simulink model "clearing_faulted_segment_travelling_Wave"  (R2018a)
settings: Solver=ode23t  StartTime=0.0  StopTime=2  MaxStep=1e-3  RelTol=1e-3
values from neighbouring files (symbols this model uses):
  AC_lim = [1.5 -1.5]    [MT_HVDC_initialize.m]
  C_pm = 10.48e-3    (= 0.01048)    [MT_HVDC_initialize.m]
  ccsc_lim = [1.0 -1.0]    [MT_HVDC_initialize.m]
  DC_lim = [1.05 -1.05]    [MT_HVDC_initialize.m]
  f = 50    [MT_HVDC_initialize.m]
  Fc = 50    [MT_HVDC_initialize.m]
  Fn_filter = 1000    [MT_HVDC_initialize.m]
  Ireg_lim_i = [1.5, -1.5]    [MT_HVDC_initialize.m]
  Ireg_lim_r = [1.5, -1.5]    [MT_HVDC_initialize.m]
  Ki_ACreg_i = 260    [MT_HVDC_initialize.m]
  Ki_ccsc = 5    [MT_HVDC_initialize.m]
  Ki_DCreg_r = 150    [MT_HVDC_initialize.m]
  Ki_Ireg_i = 200    [MT_HVDC_initialize.m]
  Ki_Ireg_r = 100    [MT_HVDC_initialize.m]
  Ki_R_inv = 150000    [MT_HVDC_initialize.m]
  Ki_R_rec = 5000    [MT_HVDC_initialize.m]
  Kp_ACreg_i = 2    [MT_HVDC_initialize.m]
  Kp_ccsc = 1    [MT_HVDC_initialize.m]
  Kp_DCreg_r = 8    [MT_HVDC_initialize.m]
  Kp_Ireg_i = 2    [MT_HVDC_initialize.m]
  Kp_Ireg_r = 2    [MT_HVDC_initialize.m]
  Kp_R_inv = 0.001    [MT_HVDC_initialize.m]
  Kp_R_rec = 0.001    [MT_HVDC_initialize.m]
  L1_pu = 0.109    [MT_HVDC_initialize.m]
  L2_pu = 0.0824    [MT_HVDC_initialize.m]
  L_arm = L_arm_pu*Z_base66/w    [MT_HVDC_initialize.m]
  L_arm_pu = 0.15    [MT_HVDC_initialize.m]
  L_int = X_int/w    [MT_HVDC_initialize.m]
  n = 50    [MT_HVDC_initialize.m]
  n2 = 50    [MT_HVDC_initialize.m]
  P_nom = 220e6    (= 220000000)    [MT_HVDC_initialize.m]
  R1_pu = 0.00206    [MT_HVDC_initialize.m]
  R2_pu = 0.00206    [MT_HVDC_initialize.m]
  R_arm = 0.03    [MT_HVDC_initialize.m]
  R_arm_pu = R_arm/Z_base66    [MT_HVDC_initialize.m]
  R_int = sqrt((z_int_400^2)/(1+xr_ratio^2))    [MT_HVDC_initialize.m]
  Rg_T1 = 40    [MT_HVDC_initialize.m]
  S1_nom = P_nom    (= 220000000)    [MT_HVDC_initialize.m]
  S2_nom = P_nom    (= 220000000)    [MT_HVDC_initialize.m]
  T_fault = 1.4    [MT_HVDC_initialize.m]
  Ts_Control = 40e-6    (= 4e-05)    [MT_HVDC_initialize.m]
  Ts_Power = 20e-6    (= 2e-05)    [MT_HVDC_initialize.m]
  V1_prim = V_prim    (= 400000)    [MT_HVDC_initialize.m]
  V1_sec = V_grid    (= 66000)    [MT_HVDC_initialize.m]
  V2_prim = V_grid    (= 66000)    [MT_HVDC_initialize.m]
  V2_sec = 18e3    (= 18000)    [MT_HVDC_initialize.m]
  V_ac_ref = 1.035    [MT_HVDC_initialize.m]
  V_grid = 66e3    (= 66000)    [MT_HVDC_initialize.m]
  V_prim = 400e3    (= 400000)    [MT_HVDC_initialize.m]
  Vc_pm_r = 0*Vdc_nom/n    (= 0)    [MT_HVDC_initialize.m]
  Vdc_nom = 135e3    (= 135000)    [MT_HVDC_initialize.m]
  w = 2*pi*f    (= 314.159265359)    [MT_HVDC_initialize.m]
  z0z1 = 0.8    [MT_HVDC_initialize.m]
  Zeta_filter = 1    [MT_HVDC_initialize.m]
undefined symbols (not defined in the file or in its folder): D1, Delta, DiscIntNeverNeededParam
libraries: powerlib x417, powerlib_meascontrol x130, simulink x84, powerlib_extras x8, simulink_extras x5
(part 6 of 17)

== system clearing_faulted_segment_travelling_Wave/MMC Converter4 ==
  g : Inport
  Current Measurement{,1..5} (6 alike) : powerlib/Measurements/Current Measurement  PhasorSimulation=off  OutputType=Complex  PSBequivalent=0
      settings: SourceProductName=Simscape Electrical
  Demux : Demux  Outputs=6
  Half-Bridge MMC Ap : Subsystem  mask(Half-Bridge MMC - Aggregate Model){n=n, C=C_pm, Vc_Initial=Vc_pm_r, Ts=Ts_Power}
      mask prompts: n "Number of power modules"; C "Capacitor value (F):"; Vc_Initial "Capacitor initial voltage (V):"; Ts "Sample time (s):"
      mask help:
      | Implement a half-bridge Modular Multilevel Converter (MMC) using a switching-function model where only one equivalent module is used to represent all power modules.
      |
      | The control signal is a two-element vector [ Nin, Nbl ], where Nin represents the number of inserted modules and Nbl represents the number of modules in the blocked-state. The output Vc (capacitor voltage) has only one element and gives the average value of the capacitors modules.
      |
      | With this aggregate model, it is assumed that capacitor voltage of all power modules are well-balanced. However, control system dynamics, converter harmonics content and circulating currents phenomena are all-well represented. The model runs a lot faster than the detailed model which uses two switching devices and one capacitor for each individual power module. This aggregate model is also well-suited for real-time simulation.
      settings: AttributesFormatString=(Aggregate model of %<n> PM)
      mask Display:
      | x1=0.0;
      | plot([0.17 0.5]+x1,[0.93 0.93])
      | plot([0.5 0.5]+x1,[0.93,0.80])
      | plot([0.5 0.38]+x1,[0.80 0.74])
      | plot([0.38 0.38]+x1,[0.80 0.62])
      | plot([0.38 0.5]+x1,[0.68 0.62])
      | plot([0.5 0.5]+x1,[0.62 0.52])
      | plot([0.45 0.5 0.43]+x1,[0.68 0.62 0.60])
      | %
      | y1=0.40-0.03;
      | plot([0.5 0.5]+x1,[0.93,0.80]-y1)
      | plot([0.5 0.38]+x1,[0.80 0.74]-y1)
      | plot([0.38 0.38]+x1,[0.80 0.62]-y1)
      | plot([0.38 0.5]+x1,[0.68 0.62]-y1)
      | plot([0.5 0.5]+x1,[0.62 0.52]-y1)
      | plot([0.45 0.5 0.43]+x1,[0.68 0.62 0.60]-y1)
      | plot([0.5 0.5]+x1,[0.2,0.10])
      | plot([0.17 0.5]+x1,[0.1 0.1])
      | %
      | plot([0.5 0.6]+x1,[0.84 0.84]+0.03)
      | plot([0.6 0.6]+x1,[0.84 0.74]+0.03)
      | plot([0.6 0.56]+x1,[0.74 0.69]+0.03)
      | plot([0.6 0.64]+x1,[0.74 0.69]+0.03)
      | plot([0.56 0.64]+x1,[0.69 0.69]+0.03)
      | plot([0.6 0.6]+x1,[0.69 0.57]+0.03)
      | plot([0.5 0.6]+x1,[0.57 0.57]+0.03)
      | plot([0.55 0.65]+x1,[0.74 0.74]+0.03)
      | %
      | y2=0.4-0.03;
      | plot([0.5 0.6]+x1,[0.84 0.84]-y2)
      | plot([0.6 0.6]+x1,[0.84 0.74]-y2)
      | plot([0.6 0.56]+x1,[0.74 0.69]-y2)
      | plot([0.6 0.64]+x1,[0.74 0.69]-y2)
      | plot([0.56 0.64]+x1,[0.69 0.69]-y2)
      | plot([0.6 0.6]+x1,[0.69 0.57]-y2)
      | plot([0.5 0.6]+x1,[0.57 0.57]-y2)
      | plot([0.55 0.65]+x1,[0.74 0.74]-y2)
      | %
      | plot([0.5 0.75]+x1,[0.53 0.53])
      | plot([0.75 0.75]+x1,[0.53 0.57])
      | plot([0.75 0.75]+x1,[0.61 0.65])
      | plot([0.75 0.75]+x1,[0.69 0.73])
      | plot([0.75 0.75]+x1,[0.77 0.81])
      | plot([0.75 0.75]+x1,[0.09 0.07])
      | plot([0.75 0.75]+x1,[0.04 0.01])
      | %
      | plot([0.34 0.34]+x1,[0.65 0.75])
      | plot([0.28 0.34]+x1,[0.7 0.7])
      | %
      | plot([0.34 0.34]+x1,[0.65 0.75]-y2)
      | plot([0.28 0.34]+x1,[0.7 0.7]-y2)
      | %
      | %Capacitor
      | plot([0.16 0.16],[0.93 0.54])
      | plot([0.16 0.16],[0.47 0.10])
      | plot([0.04 0.27],[0.54 0.54])
      | plot([0.04 0.27],[0.47 0.47])
      | %
      | plot([0.5 0.75],[0.1 0.1])
      | % text(0.78,0.5,'1')
      | % text(0.78,0.12,'2')
      | %
      | color('blue')
      | port_label('input',1,'N')
  Half-Bridge MMC Ap1 : Subsystem  mask(Half-Bridge MMC - Aggregate Model){n=n, C=C_pm, Vc_Initial=Vc_pm_r, Ts=Ts_Power}
      mask prompts: n "Number of power modules"; C "Capacitor value (F):"; Vc_Initial "Capacitor initial voltage (V):"; Ts "Sample time (s):"
      mask help:
      | Implement a half-bridge Modular Multilevel Converter (MMC) using a switching-function model where only one equivalent module is used to represent all power modules.
      |
      | The control signal is a two-element vector [ Nin, Nbl ], where Nin represents the number of inserted modules and Nbl represents the number of modules in the blocked-state. The output Vc (capacitor voltage) has only one element and gives the average value of the capacitors modules.
      |
      | With this aggregate model, it is assumed that capacitor voltage of all power modules are well-balanced. However, control system dynamics, converter harmonics content and circulating currents phenomena are all-well represented. The model runs a lot faster than the detailed model which uses two switching devices and one capacitor for each individual power module. This aggregate model is also well-suited for real-time simulation.
      settings: AttributesFormatString=(Aggregate model of %<n> PM)
      mask Display:
      | x1=0.0;
      | plot([0.17 0.5]+x1,[0.93 0.93])
      | plot([0.5 0.5]+x1,[0.93,0.80])
      | plot([0.5 0.38]+x1,[0.80 0.74])
      | plot([0.38 0.38]+x1,[0.80 0.62])
      | plot([0.38 0.5]+x1,[0.68 0.62])
      | plot([0.5 0.5]+x1,[0.62 0.52])
      | plot([0.45 0.5 0.43]+x1,[0.68 0.62 0.60])
      | %
      | y1=0.40-0.03;
      | plot([0.5 0.5]+x1,[0.93,0.80]-y1)
      | plot([0.5 0.38]+x1,[0.80 0.74]-y1)
      | plot([0.38 0.38]+x1,[0.80 0.62]-y1)
      | plot([0.38 0.5]+x1,[0.68 0.62]-y1)
      | plot([0.5 0.5]+x1,[0.62 0.52]-y1)
      | plot([0.45 0.5 0.43]+x1,[0.68 0.62 0.60]-y1)
      | plot([0.5 0.5]+x1,[0.2,0.10])
      | plot([0.17 0.5]+x1,[0.1 0.1])
      | %
      | plot([0.5 0.6]+x1,[0.84 0.84]+0.03)
      | plot([0.6 0.6]+x1,[0.84 0.74]+0.03)
      | plot([0.6 0.56]+x1,[0.74 0.69]+0.03)
      | plot([0.6 0.64]+x1,[0.74 0.69]+0.03)
      | plot([0.56 0.64]+x1,[0.69 0.69]+0.03)
      | plot([0.6 0.6]+x1,[0.69 0.57]+0.03)
      | plot([0.5 0.6]+x1,[0.57 0.57]+0.03)
      | plot([0.55 0.65]+x1,[0.74 0.74]+0.03)
      | %
      | y2=0.4-0.03;
      | plot([0.5 0.6]+x1,[0.84 0.84]-y2)
      | plot([0.6 0.6]+x1,[0.84 0.74]-y2)
      | plot([0.6 0.56]+x1,[0.74 0.69]-y2)
      | plot([0.6 0.64]+x1,[0.74 0.69]-y2)
      | plot([0.56 0.64]+x1,[0.69 0.69]-y2)
      | plot([0.6 0.6]+x1,[0.69 0.57]-y2)
      | plot([0.5 0.6]+x1,[0.57 0.57]-y2)
      | plot([0.55 0.65]+x1,[0.74 0.74]-y2)
      | %
      | plot([0.5 0.75]+x1,[0.53 0.53])
      | plot([0.75 0.75]+x1,[0.53 0.57])
      | plot([0.75 0.75]+x1,[0.61 0.65])
      | plot([0.75 0.75]+x1,[0.69 0.73])
      | plot([0.75 0.75]+x1,[0.77 0.81])
      | plot([0.75 0.75]+x1,[0.09 0.07])
      | plot([0.75 0.75]+x1,[0.04 0.01])
      | %
      | plot([0.34 0.34]+x1,[0.65 0.75])
      | plot([0.28 0.34]+x1,[0.7 0.7])
      | %
      | plot([0.34 0.34]+x1,[0.65 0.75]-y2)
      | plot([0.28 0.34]+x1,[0.7 0.7]-y2)
      | %
      | %Capacitor
      | plot([0.16 0.16],[0.93 0.54])
      | plot([0.16 0.16],[0.47 0.10])
      | plot([0.04 0.27],[0.54 0.54])
      | plot([0.04 0.27],[0.47 0.47])
      | %
      | plot([0.5 0.75],[0.1 0.1])
      | % text(0.78,0.5,'1')
      | % text(0.78,0.12,'2')
      | %
      | color('blue')
      | port_label('input',1,'N')
  Half-Bridge MMC Ap2 : Subsystem  mask(Half-Bridge MMC - Aggregate Model){n=n, C=C_pm, Vc_Initial=Vc_pm_r, Ts=Ts_Power}
      mask prompts: n "Number of power modules"; C "Capacitor value (F):"; Vc_Initial "Capacitor initial voltage (V):"; Ts "Sample time (s):"
      mask help:
      | Implement a half-bridge Modular Multilevel Converter (MMC) using a switching-function model where only one equivalent module is used to represent all power modules.
      |
      | The control signal is a two-element vector [ Nin, Nbl ], where Nin represents the number of inserted modules and Nbl represents the number of modules in the blocked-state. The output Vc (capacitor voltage) has only one element and gives the average value of the capacitors modules.
      |
      | With this aggregate model, it is assumed that capacitor voltage of all power modules are well-balanced. However, control system dynamics, converter harmonics content and circulating currents phenomena are all-well represented. The model runs a lot faster than the detailed model which uses two switching devices and one capacitor for each individual power module. This aggregate model is also well-suited for real-time simulation.
      settings: AttributesFormatString=(Aggregate model of %<n> PM)
      mask Display:
      | x1=0.0;
      | plot([0.17 0.5]+x1,[0.93 0.93])
      | plot([0.5 0.5]+x1,[0.93,0.80])
      | plot([0.5 0.38]+x1,[0.80 0.74])
      | plot([0.38 0.38]+x1,[0.80 0.62])
      | plot([0.38 0.5]+x1,[0.68 0.62])
      | plot([0.5 0.5]+x1,[0.62 0.52])
      | plot([0.45 0.5 0.43]+x1,[0.68 0.62 0.60])
      | %
      | y1=0.40-0.03;
      | plot([0.5 0.5]+x1,[0.93,0.80]-y1)
      | plot([0.5 0.38]+x1,[0.80 0.74]-y1)
      | plot([0.38 0.38]+x1,[0.80 0.62]-y1)
      | plot([0.38 0.5]+x1,[0.68 0.62]-y1)
      | plot([0.5 0.5]+x1,[0.62 0.52]-y1)
      | plot([0.45 0.5 0.43]+x1,[0.68 0.62 0.60]-y1)
      | plot([0.5 0.5]+x1,[0.2,0.10])
      | plot([0.17 0.5]+x1,[0.1 0.1])
      | %
      | plot([0.5 0.6]+x1,[0.84 0.84]+0.03)
      | plot([0.6 0.6]+x1,[0.84 0.74]+0.03)
      | plot([0.6 0.56]+x1,[0.74 0.69]+0.03)
      | plot([0.6 0.64]+x1,[0.74 0.69]+0.03)
      | plot([0.56 0.64]+x1,[0.69 0.69]+0.03)
      | plot([0.6 0.6]+x1,[0.69 0.57]+0.03)
      | plot([0.5 0.6]+x1,[0.57 0.57]+0.03)
      | plot([0.55 0.65]+x1,[0.74 0.74]+0.03)
      | %
      | y2=0.4-0.03;
      | plot([0.5 0.6]+x1,[0.84 0.84]-y2)
      | plot([0.6 0.6]+x1,[0.84 0.74]-y2)
      | plot([0.6 0.56]+x1,[0.74 0.69]-y2)
      | plot([0.6 0.64]+x1,[0.74 0.69]-y2)
      | plot([0.56 0.64]+x1,[0.69 0.69]-y2)
      | plot([0.6 0.6]+x1,[0.69 0.57]-y2)
      | plot([0.5 0.6]+x1,[0.57 0.57]-y2)
      | plot([0.55 0.65]+x1,[0.74 0.74]-y2)
      | %
      | plot([0.5 0.75]+x1,[0.53 0.53])
      | plot([0.75 0.75]+x1,[0.53 0.57])
      | plot([0.75 0.75]+x1,[0.61 0.65])
      | plot([0.75 0.75]+x1,[0.69 0.73])
      | plot([0.75 0.75]+x1,[0.77 0.81])
      | plot([0.75 0.75]+x1,[0.09 0.07])
      | plot([0.75 0.75]+x1,[0.04 0.01])
      | %
      | plot([0.34 0.34]+x1,[0.65 0.75])
      | plot([0.28 0.34]+x1,[0.7 0.7])
      | %
      | plot([0.34 0.34]+x1,[0.65 0.75]-y2)
      | plot([0.28 0.34]+x1,[0.7 0.7]-y2)
      | %
      | %Capacitor
      | plot([0.16 0.16],[0.93 0.54])
      | plot([0.16 0.16],[0.47 0.10])
      | plot([0.04 0.27],[0.54 0.54])
      | plot([0.04 0.27],[0.47 0.47])
      | %
      | plot([0.5 0.75],[0.1 0.1])
      | % text(0.78,0.5,'1')
      | % text(0.78,0.12,'2')
      | %
      | color('blue')
      | port_label('input',1,'N')
  Half-Bridge MMC Ap3 : Subsystem  mask(Half-Bridge MMC - Aggregate Model){n=n, C=C_pm, Vc_Initial=Vc_pm_r, Ts=Ts_Power}
      mask prompts: n "Number of power modules"; C "Capacitor value (F):"; Vc_Initial "Capacitor initial voltage (V):"; Ts "Sample time (s):"
      mask help:
      | Implement a half-bridge Modular Multilevel Converter (MMC) using a switching-function model where only one equivalent module is used to represent all power modules.
      |
      | The control signal is a two-element vector [ Nin, Nbl ], where Nin represents the number of inserted modules and Nbl represents the number of modules in the blocked-state. The output Vc (capacitor voltage) has only one element and gives the average value of the capacitors modules.
      |
      | With this aggregate model, it is assumed that capacitor voltage of all power modules are well-balanced. However, control system dynamics, converter harmonics content and circulating currents phenomena are all-well represented. The model runs a lot faster than the detailed model which uses two switching devices and one capacitor for each individual power module. This aggregate model is also well-suited for real-time simulation.
      settings: AttributesFormatString=(Aggregate model of %<n> PM)
      mask Display:
      | x1=0.0;
      | plot([0.17 0.5]+x1,[0.93 0.93])
      | plot([0.5 0.5]+x1,[0.93,0.80])
      | plot([0.5 0.38]+x1,[0.80 0.74])
      | plot([0.38 0.38]+x1,[0.80 0.62])
      | plot([0.38 0.5]+x1,[0.68 0.62])
      | plot([0.5 0.5]+x1,[0.62 0.52])
      | plot([0.45 0.5 0.43]+x1,[0.68 0.62 0.60])
      | %
      | y1=0.40-0.03;
      | plot([0.5 0.5]+x1,[0.93,0.80]-y1)
      | plot([0.5 0.38]+x1,[0.80 0.74]-y1)
      | plot([0.38 0.38]+x1,[0.80 0.62]-y1)
      | plot([0.38 0.5]+x1,[0.68 0.62]-y1)
      | plot([0.5 0.5]+x1,[0.62 0.52]-y1)
      | plot([0.45 0.5 0.43]+x1,[0.68 0.62 0.60]-y1)
      | plot([0.5 0.5]+x1,[0.2,0.10])
      | plot([0.17 0.5]+x1,[0.1 0.1])
      | %
      | plot([0.5 0.6]+x1,[0.84 0.84]+0.03)
      | plot([0.6 0.6]+x1,[0.84 0.74]+0.03)
      | plot([0.6 0.56]+x1,[0.74 0.69]+0.03)
      | plot([0.6 0.64]+x1,[0.74 0.69]+0.03)
      | plot([0.56 0.64]+x1,[0.69 0.69]+0.03)
      | plot([0.6 0.6]+x1,[0.69 0.57]+0.03)
      | plot([0.5 0.6]+x1,[0.57 0.57]+0.03)
      | plot([0.55 0.65]+x1,[0.74 0.74]+0.03)
      | %
      | y2=0.4-0.03;
      | plot([0.5 0.6]+x1,[0.84 0.84]-y2)
      | plot([0.6 0.6]+x1,[0.84 0.74]-y2)
      | plot([0.6 0.56]+x1,[0.74 0.69]-y2)
      | plot([0.6 0.64]+x1,[0.74 0.69]-y2)
      | plot([0.56 0.64]+x1,[0.69 0.69]-y2)
      | plot([0.6 0.6]+x1,[0.69 0.57]-y2)
      | plot([0.5 0.6]+x1,[0.57 0.57]-y2)
      | plot([0.55 0.65]+x1,[0.74 0.74]-y2)
      | %
      | plot([0.5 0.75]+x1,[0.53 0.53])
      | plot([0.75 0.75]+x1,[0.53 0.57])
      | plot([0.75 0.75]+x1,[0.61 0.65])
      | plot([0.75 0.75]+x1,[0.69 0.73])
      | plot([0.75 0.75]+x1,[0.77 0.81])
      | plot([0.75 0.75]+x1,[0.09 0.07])
      | plot([0.75 0.75]+x1,[0.04 0.01])
      | %
      | plot([0.34 0.34]+x1,[0.65 0.75])
      | plot([0.28 0.34]+x1,[0.7 0.7])
      | %
      | plot([0.34 0.34]+x1,[0.65 0.75]-y2)
      | plot([0.28 0.34]+x1,[0.7 0.7]-y2)
      | %
      | %Capacitor
      | plot([0.16 0.16],[0.93 0.54])
      | plot([0.16 0.16],[0.47 0.10])
      | plot([0.04 0.27],[0.54 0.54])
      | plot([0.04 0.27],[0.47 0.47])
      | %
      | plot([0.5 0.75],[0.1 0.1])
      | % text(0.78,0.5,'1')
      | % text(0.78,0.12,'2')
      | %
      | color('blue')
      | port_label('input',1,'N')
  Half-Bridge MMC Ap4 : Subsystem  mask(Half-Bridge MMC - Aggregate Model){n=n, C=C_pm, Vc_Initial=Vc_pm_r, Ts=Ts_Power}
      mask prompts: n "Number of power modules"; C "Capacitor value (F):"; Vc_Initial "Capacitor initial voltage (V):"; Ts "Sample time (s):"
      mask help:
      | Implement a half-bridge Modular Multilevel Converter (MMC) using a switching-function model where only one equivalent module is used to represent all power modules.
      |
      | The control signal is a two-element vector [ Nin, Nbl ], where Nin represents the number of inserted modules and Nbl represents the number of modules in the blocked-state. The output Vc (capacitor voltage) has only one element and gives the average value of the capacitors modules.
      |
      | With this aggregate model, it is assumed that capacitor voltage of all power modules are well-balanced. However, control system dynamics, converter harmonics content and circulating currents phenomena are all-well represented. The model runs a lot faster than the detailed model which uses two switching devices and one capacitor for each individual power module. This aggregate model is also well-suited for real-time simulation.
      settings: AttributesFormatString=(Aggregate model of %<n> PM)
      mask Display:
      | x1=0.0;
      | plot([0.17 0.5]+x1,[0.93 0.93])
      | plot([0.5 0.5]+x1,[0.93,0.80])
      | plot([0.5 0.38]+x1,[0.80 0.74])
      | plot([0.38 0.38]+x1,[0.80 0.62])
      | plot([0.38 0.5]+x1,[0.68 0.62])
      | plot([0.5 0.5]+x1,[0.62 0.52])
      | plot([0.45 0.5 0.43]+x1,[0.68 0.62 0.60])
      | %
      | y1=0.40-0.03;
      | plot([0.5 0.5]+x1,[0.93,0.80]-y1)
      | plot([0.5 0.38]+x1,[0.80 0.74]-y1)
      | plot([0.38 0.38]+x1,[0.80 0.62]-y1)
      | plot([0.38 0.5]+x1,[0.68 0.62]-y1)
      | plot([0.5 0.5]+x1,[0.62 0.52]-y1)
      | plot([0.45 0.5 0.43]+x1,[0.68 0.62 0.60]-y1)
      | plot([0.5 0.5]+x1,[0.2,0.10])
      | plot([0.17 0.5]+x1,[0.1 0.1])
      | %
      | plot([0.5 0.6]+x1,[0.84 0.84]+0.03)
      | plot([0.6 0.6]+x1,[0.84 0.74]+0.03)
      | plot([0.6 0.56]+x1,[0.74 0.69]+0.03)
      | plot([0.6 0.64]+x1,[0.74 0.69]+0.03)
      | plot([0.56 0.64]+x1,[0.69 0.69]+0.03)
      | plot([0.6 0.6]+x1,[0.69 0.57]+0.03)
      | plot([0.5 0.6]+x1,[0.57 0.57]+0.03)
      | plot([0.55 0.65]+x1,[0.74 0.74]+0.03)
      | %
      | y2=0.4-0.03;
      | plot([0.5 0.6]+x1,[0.84 0.84]-y2)
      | plot([0.6 0.6]+x1,[0.84 0.74]-y2)
      | plot([0.6 0.56]+x1,[0.74 0.69]-y2)
      | plot([0.6 0.64]+x1,[0.74 0.69]-y2)
      | plot([0.56 0.64]+x1,[0.69 0.69]-y2)
      | plot([0.6 0.6]+x1,[0.69 0.57]-y2)
      | plot([0.5 0.6]+x1,[0.57 0.57]-y2)
      | plot([0.55 0.65]+x1,[0.74 0.74]-y2)
      | %
      | plot([0.5 0.75]+x1,[0.53 0.53])
      | plot([0.75 0.75]+x1,[0.53 0.57])
      | plot([0.75 0.75]+x1,[0.61 0.65])
      | plot([0.75 0.75]+x1,[0.69 0.73])
      | plot([0.75 0.75]+x1,[0.77 0.81])
      | plot([0.75 0.75]+x1,[0.09 0.07])
      | plot([0.75 0.75]+x1,[0.04 0.01])
      | %
      | plot([0.34 0.34]+x1,[0.65 0.75])
      | plot([0.28 0.34]+x1,[0.7 0.7])
      | %
      | plot([0.34 0.34]+x1,[0.65 0.75]-y2)
      | plot([0.28 0.34]+x1,[0.7 0.7]-y2)
      | %
      | %Capacitor
      | plot([0.16 0.16],[0.93 0.54])
      | plot([0.16 0.16],[0.47 0.10])
      | plot([0.04 0.27],[0.54 0.54])
      | plot([0.04 0.27],[0.47 0.47])
      | %
      | plot([0.5 0.75],[0.1 0.1])
      | % text(0.78,0.5,'1')
      | % text(0.78,0.12,'2')
      | %
      | color('blue')
      | port_label('input',1,'N')
  Half-Bridge MMC Ap5 : Subsystem  mask(Half-Bridge MMC - Aggregate Model){n=n, C=C_pm, Vc_Initial=Vc_pm_r, Ts=Ts_Power}
      mask prompts: n "Number of power modules"; C "Capacitor value (F):"; Vc_Initial "Capacitor initial voltage (V):"; Ts "Sample time (s):"
      mask help:
      | Implement a half-bridge Modular Multilevel Converter (MMC) using a switching-function model where only one equivalent module is used to represent all power modules.
      |
      | The control signal is a two-element vector [ Nin, Nbl ], where Nin represents the number of inserted modules and Nbl represents the number of modules in the blocked-state. The output Vc (capacitor voltage) has only one element and gives the average value of the capacitors modules.
      |
      | With this aggregate model, it is assumed that capacitor voltage of all power modules are well-balanced. However, control system dynamics, converter harmonics content and circulating currents phenomena are all-well represented. The model runs a lot faster than the detailed model which uses two switching devices and one capacitor for each individual power module. This aggregate model is also well-suited for real-time simulation.
      settings: AttributesFormatString=(Aggregate model of %<n> PM)
      mask Display:
      | x1=0.0;
      | plot([0.17 0.5]+x1,[0.93 0.93])
      | plot([0.5 0.5]+x1,[0.93,0.80])
      | plot([0.5 0.38]+x1,[0.80 0.74])
      | plot([0.38 0.38]+x1,[0.80 0.62])
      | plot([0.38 0.5]+x1,[0.68 0.62])
      | plot([0.5 0.5]+x1,[0.62 0.52])
      | plot([0.45 0.5 0.43]+x1,[0.68 0.62 0.60])
      | %
      | y1=0.40-0.03;
      | plot([0.5 0.5]+x1,[0.93,0.80]-y1)
      | plot([0.5 0.38]+x1,[0.80 0.74]-y1)
      | plot([0.38 0.38]+x1,[0.80 0.62]-y1)
      | plot([0.38 0.5]+x1,[0.68 0.62]-y1)
      | plot([0.5 0.5]+x1,[0.62 0.52]-y1)
      | plot([0.45 0.5 0.43]+x1,[0.68 0.62 0.60]-y1)
      | plot([0.5 0.5]+x1,[0.2,0.10])
      | plot([0.17 0.5]+x1,[0.1 0.1])
      | %
      | plot([0.5 0.6]+x1,[0.84 0.84]+0.03)
      | plot([0.6 0.6]+x1,[0.84 0.74]+0.03)
      | plot([0.6 0.56]+x1,[0.74 0.69]+0.03)
      | plot([0.6 0.64]+x1,[0.74 0.69]+0.03)
      | plot([0.56 0.64]+x1,[0.69 0.69]+0.03)
      | plot([0.6 0.6]+x1,[0.69 0.57]+0.03)
      | plot([0.5 0.6]+x1,[0.57 0.57]+0.03)
      | plot([0.55 0.65]+x1,[0.74 0.74]+0.03)
      | %
      | y2=0.4-0.03;
      | plot([0.5 0.6]+x1,[0.84 0.84]-y2)
      | plot([0.6 0.6]+x1,[0.84 0.74]-y2)
      | plot([0.6 0.56]+x1,[0.74 0.69]-y2)
      | plot([0.6 0.64]+x1,[0.74 0.69]-y2)
      | plot([0.56 0.64]+x1,[0.69 0.69]-y2)
      | plot([0.6 0.6]+x1,[0.69 0.57]-y2)
      | plot([0.5 0.6]+x1,[0.57 0.57]-y2)
      | plot([0.55 0.65]+x1,[0.74 0.74]-y2)
      | %
      | plot([0.5 0.75]+x1,[0.53 0.53])
      | plot([0.75 0.75]+x1,[0.53 0.57])
      | plot([0.75 0.75]+x1,[0.61 0.65])
      | plot([0.75 0.75]+x1,[0.69 0.73])
      | plot([0.75 0.75]+x1,[0.77 0.81])
      | plot([0.75 0.75]+x1,[0.09 0.07])
      | plot([0.75 0.75]+x1,[0.04 0.01])
      | %
      | plot([0.34 0.34]+x1,[0.65 0.75])
      | plot([0.28 0.34]+x1,[0.7 0.7])
      | %
      | plot([0.34 0.34]+x1,[0.65 0.75]-y2)
      | plot([0.28 0.34]+x1,[0.7 0.7]-y2)
      | %
      | %Capacitor
      | plot([0.16 0.16],[0.93 0.54])
      | plot([0.16 0.16],[0.47 0.10])
      | plot([0.04 0.27],[0.54 0.54])
      | plot([0.04 0.27],[0.47 0.47])
      | %
      | plot([0.5 0.75],[0.1 0.1])
      | % text(0.78,0.5,'1')
      | % text(0.78,0.12,'2')
      | %
      | color('blue')
      | port_label('input',1,'N')
  Mux : Mux  Inputs=6
  Mux1 : Mux  Inputs=6
  Series RLC Branch1 : powerlib/Elements/Series RLC Branch  LConnTagsString=__new0  RConnTagsString=__new0  BranchType=L  Resistance=R_arm  Inductance=L_arm  SetiL0=off  InitialCurrent=0  Capacitance=1e-6  Setx0=off  InitialVoltage=0  Measurements=None
      settings: SourceProductName=Simscape Electrical
  Series RLC Branch{2..6} (5 alike) : powerlib/Elements/Series RLC Branch  LConnTagsString=__new0  RConnTagsString=__new0  BranchType=RL  Resistance=R_arm  Inductance=L_arm  SetiL0=off  InitialCurrent=0  Capacitance=1e-6  Setx0=off  InitialVoltage=0  Measurements=None
      settings: SourceProductName=Simscape Electrical
  Series RLC Branch7 : powerlib/Elements/Series RLC Branch  LConnTagsString=__new0  RConnTagsString=__new0  BranchType=R  Resistance=R_arm  Inductance=L_arm  SetiL0=off  InitialCurrent=0  Capacitance=1e-6  Setx0=off  InitialVoltage=0  Measurements=None
      settings: SourceProductName=Simscape Electrical
  V_a : PMIOPort  Tag=PMCPort  Side=Left
  V_b : PMIOPort  Tag=PMCPort  Port=2  Side=Left
  V_c : PMIOPort  Tag=PMCPort  Port=3  Side=Left
  Vdc + : PMIOPort  Tag=PMCPort  Port=4  Side=Right
  Vdc - : PMIOPort  Tag=PMCPort  Port=5  Side=Right
  Vc : Outport
  I_arm : Outport  Port=2
  wires:
  Demux/6 -> [g6]
  Demux/5 -> [g5]
  Demux/4 -> [g4]
  Demux/3 -> [g3]
  Demux/2 -> [g2]
  Demux/1 -> [g1]
  Half-Bridge MMC Ap/1(Vc) -> [Vc1]
  Half-Bridge MMC Ap5/1(Vc) -> [Vc6]
  Half-Bridge MMC Ap3/1(Vc) -> [Vc2]
  Half-Bridge MMC Ap4/1(Vc) -> [Vc5]
  [Icu] -> Mux1/5
  [Ibl] -> Mux1/4
  [Icl] -> Mux1/6
  [Ial] -> Mux1/2
  [Iau] -> Mux1/1
  Mux1/1 -> I_arm/1
  [Ibu] -> Mux1/3
  Current Measurement2/1 -> [Ibu]
  Current Measurement5/1 -> [Icl]
  Current Measurement3/1 -> [Icu]
  Current Measurement4/1 -> [Ibl]
  Current Measurement/1 -> [Iau]
  Current Measurement1/1 -> [Ial]
  [Vc5] -> Mux/5
  Mux/1 -> Vc/1
  [Vc4] -> Mux/4
  [Vc1] -> Mux/1
  [Vc6] -> Mux/6
  [Vc3] -> Mux/3
  [g5] -> Half-Bridge MMC Ap1/1(g)
  [g1] -> Half-Bridge MMC Ap/1(g)
  [g4] -> Half-Bridge MMC Ap3/1(g)
  [g3] -> Half-Bridge MMC Ap4/1(g)
  [g2] -> Half-Bridge MMC Ap2/1(g)
  [g6] -> Half-Bridge MMC Ap5/1(g)
  g/1 -> Demux/1
  [Vc2] -> Mux/2
  Half-Bridge MMC Ap1/1(Vc) -> [Vc4]
  Half-Bridge MMC Ap2/1(Vc) -> [Vc3]
  connections:
  Half-Bridge MMC Ap1/LConn1 -- Current Measurement4/RConn1
  Half-Bridge MMC Ap5/LConn1 -- Current Measurement5/RConn1
  Half-Bridge MMC Ap2/LConn2 -- Current Measurement2/LConn1
  Half-Bridge MMC Ap4/LConn2 -- Current Measurement3/LConn1
  Vdc -/RConn1 -- Half-Bridge MMC Ap3/LConn2 -- Half-Bridge MMC Ap5/LConn2 -- Half-Bridge MMC Ap1/LConn2
  Half-Bridge MMC Ap3/LConn1 -- Current Measurement1/RConn1
  V_b/RConn1 -- Series RLC Branch2/RConn1 -- Series RLC Branch4/LConn1
  Series RLC Branch1/LConn1 -- Series RLC Branch7/RConn1
  Series RLC Branch3/RConn1 -- Current Measurement1/LConn1
  V_c/RConn1 -- Series RLC Branch5/LConn1 -- Series RLC Branch6/RConn1
  V_a/RConn1 -- Series RLC Branch1/RConn1 -- Series RLC Branch3/LConn1
  Series RLC Branch2/LConn1 -- Current Measurement2/RConn1
  Series RLC Branch4/RConn1 -- Current Measurement4/LConn1
  Current Measurement5/LConn1 -- Series RLC Branch5/RConn1
  Series RLC Branch6/LConn1 -- Current Measurement3/RConn1
  Vdc +/RConn1 -- Half-Bridge MMC Ap/LConn1 -- Half-Bridge MMC Ap4/LConn1 -- Half-Bridge MMC Ap2/LConn1
  Current Measurement/LConn1 -- Half-Bridge MMC Ap/LConn2
  Series RLC Branch7/LConn1 -- Current Measurement/RConn1

== system clearing_faulted_segment_travelling_Wave/Model Information ==
  note: References
      | [1] T. E. Slettbakk. “Development of a Power Quality Conditioning System for Particle Accelerators”.
      | Norwegian University of Science and Technology & CERN, 2019.
      |
      | [2] Georgia Tech, M. Saeedifard. “Multilevel Converters for Medium/High-
      | Power Applications”, 2018. [Online course]. Available: https://www.edx.org/
      | course/gt-multilevel-converters-for-mediumhigh-power-applications.
      |
      | [3] Cigré working group B4.57. “Guide for the Development of Models for HVDC Con-
      | verters in a HVDC Grid”. Technical Brochure 604, 2014.
      |
      | [4] P. Giroux. “SimPowerSystems Model of a 1000-MW HVDC-MMC Interconnection.”, 2015.
      | [Online]. Available: https://ch.mathworks.com/matlabcentral/fileexchange/54506-s
      | impowersystems-model-of-a-1000-mw-hvdc-mmc-interconnection
      |
      | [5] M. Saeedifard and R. Iravani. “Dynamic Performance of a Modular Multilevel Back-
      | to-Back HVDC System”. IEEE Transactions on Power Delivery, 2010.
      |
      | [6] C. Du, M. H. J. Bollen, and E. Agneholm. “A New Control Strategy of a VSC –
      | HVDC System for High-Quality Supply of Industrial Plants”. IEEE Transactions on
      | Power Delivery, 22(4):2386–2394, 2007.
      |
      | [7] R.Z. Chai et al. “Control Strategies of MMC-HVDC Connected to Passive Networks”. IEEE
      | International Conference “TENCON”, 2013.
      |
      | [8] N. Geddada, A. Ukil, and Y. M. Yeap. “Circulating Current Controller in dq Ref-
      | erence Frame for MMC Based HVDC System”. In IECON 2016 - 42nd Annual
      | Conference of the IEEE Industrial Electronics Society, pages 3288–3293, 2016.
      |
      | [9] J. Jia, G. Yang, and A. Nielsen. “Fault Analysis Method Considering Dual-Sequence
      | Current Control of VSCs under Unbalanced Faults”. Energies, 11(7), 2018.
      |
      | [10] A. Timofejevs et al. “Control of Transformerless MMC-HVDC During Asymmetric
      | Grid Faults”. In IECON 2013 - 39th Annual Conference of the IEEE Industrial
      | Electronics Society, pages 2016–2021, 2013.
      |
      | [11] Hydro-Québec. “SimPowerSystem for Use with Simulink”. TransÉnergieTechnologies
      | Inc., 2003.
      |
      | [12] K. Sharifabadi et al. “Design, Control, and Application of Modular Multilevel Con-
      | verters for HVDC Transmission Systems”. John Wiley & Sons Inc., 2016.
  note: The Back-to-Back HVDC Modular Multilevel
      | Converter for Passive Networks – Simulation Model
      |
      | Tony Endré Slettbakk – tony.slettbakk@gmail.com - CERN
      |
      | Purpose of the model
      | The model was developed through the work of the bachelor’s thesis [1] conducted at CERN in 2018, as part of the technical student program together with the Norwegian University of Science and Technology (NTNU). The thesis is titled “Development of a Power Quality Conditioning System for Particle Accelerators”. The model is used to prove the feasibility of the back-to-back HVDC converter for transient voltage dip mitigation, using the modular multilevel topology. The voltage dips are mitigated using internal energy stored in the submodule capacitors, together with extracting maximum allowed current from the grid. The potential for such a system is large, as today’s particle accelerators experience issued with transient voltage dips. Protection against this is of importance for future particle accelerators of even larger dimensions.
      | Development process
      | The model was developed in the MATLAB & SIMULINK environment, using the SimPower electrical systems. The development process started from scratch, with only basic personal experience in power electronics and simulation. Estimated time to gain knowledge of the topology and control system is around 300 hours. Time spend on the simulation model in building, refinement and validation is estimated to over 200 hours.
      | Basic knowledge of modular multilevel converters is based on the course presented in [2], while more advanced knowledge was obtained from various international publications presented in IEEE Explorer, and through technical brochures from Cigré, especially [3].
      | The modelling technique for this simulation is based on the example model of IREQ Quebec [4], and other various examples from Mathworks inc, available online. The simulation model was developed with its control system based on many separate publications and guidelines.
      | User guide
      | The model
      | The simulation model comes in two files. The first is a Matlab code ‘.m’-file, initializing most of the parameters used for simulation, used for easy access for modifications. The other file is the Simulink model ‘.slx’ file, containing the complete model. Before simulation can start, the initialization file must be ran.
      | The model is the back-to-back HVDC modular multilevel converter supplying a passive network with power. For the initial settings, the MMC rectifier and inverter is identical, and is of 51 levels. Connection voltage is 66 kV. DC voltage is 135 kV at a steady state modulation index of ~0.8. Rating of the converter is 220 MVA.
      | The control system comes in two variants. The default one is the synchronous reference frame (SRF), used for the thesis report. The dual synchronous reference frame (DSRF) is included as a variant for both rectifier and inverter control, and can be selected manually for the simulation if needed.
      | Included in the control system is the circulating current suppression controller (CCSC), operating in dq0 frame. A zero-sequence suppression controller is also included, operating with proportional-resonant (PR) controller. This is used for simulation cases where the connection transformers does not isolate the zero sequence currents from flowing. (wye-wye normally).
      | The model employs the aggregated modelling strategy for modular multilevel converter, which has the goal of increasing the computational efficiency of the model, while keeping the necessary dynamics and details. For the MMC, every submodule capacitors of one arm is modelled as a common virtual capacitor, which in physical terms means that the model assumes a perfect capacitor voltage balancing. This is only a physical property addressed in practical design, and does not affect the results of the simulation.
      | The ideology of the model is to be interactive, with ease of changing parameters. Based on this, the model can be edited with the script to simulate any levels of the MMC, presented by ‘n’ and ‘n2’ in the script, so that rectifier and inverter can operate with different amount of levels as well. The parameters that are not available in the .m-file, is usually accessible on the front-panel of the simulation model (overview-page). This is mostly the sequencing of events occurring in the model, such as control systems being enabled, load switching, etc.
      | Steady state and start-up
      | The demonstration (default settings) of the model is set to simulate start-up and charging of the converter. This is initiated through several steps from controlling breakers to enabling control systems and setting control references. It is possible to start from steady state by setting the initial submodule capacitor voltages, and remove start-up procedures.
      | Voltage dip mitigation and energy storage validation
      | The converter is initially dimensioned with a total energy of 22.9 MJ, resulting in an energy of 104 kJ/MVA of the back-to-back rating, or 52 kJ/MVA in each of the rectifier and inverter. The submodule energy is dimensioned to 38.2 kJ. This is sufficient to mitigate a symmetrical voltage dip of three phases, -50% magnitude and duration of 75ms or any equivalent, for example a unsymmetrical single-phase dip of -75% and duration of 150ms.
      | Voltage dips are simulated in the AC network source, forcing a lower voltage magnitude for a determined duration and returning to normal source operation when commanded. Both symmetrical and unsymmetrical voltage dips can be simulated.
      |
      | Fault scenarios
      | Several fault scenarios beyond voltage dips can be simulated in this model. Of this is the:
      | Ø DC bus pole-pole fault
      | Ø DC bus pole-ground fault
      | Ø Load network short circuit
      | Ø AC transmission network short circuit
      | Ø Phase to pole short circuit between AC and DC side
      | These scenarios can be triggered trough the “three-phase fault”-block in Simulink, or through breakers closing and opening at a chosen time, and is not included by default in the model.
      | Faults such as short circuit in the individual module, as well as flashover fault (between two converter arms) cannot be simulated in this model, as it employs the aggregated modelling strategy where only the whole converter arm is available.
      | Final words
      | This simulation model is a result of many publications and references, given in the reference list. Many of these references has acted as a general inspiration for the technological knowledge of MMC’s, and their control systems.

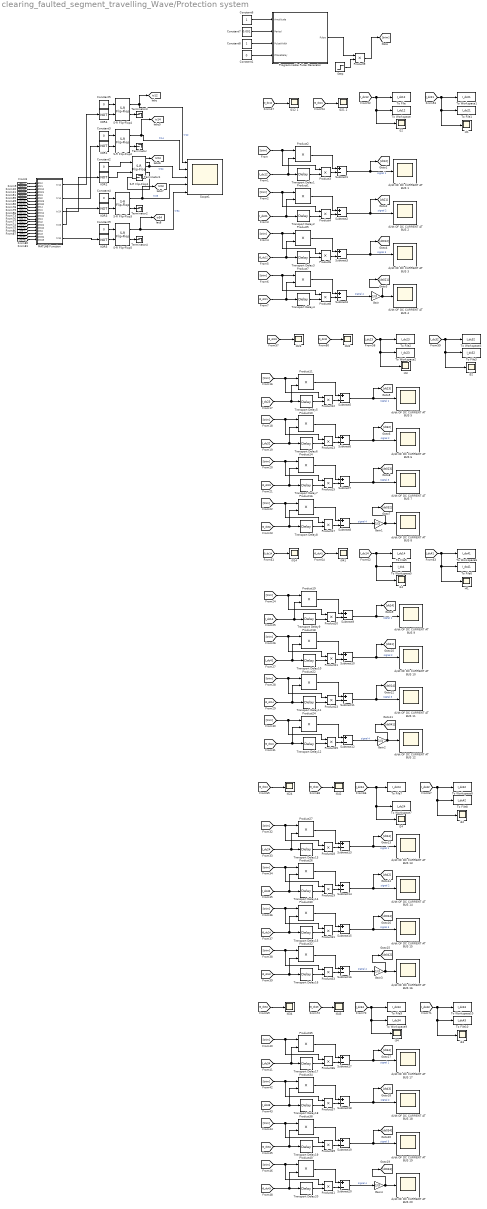
== system clearing_faulted_segment_travelling_Wave/Protection system ==
  Constant1 : Constant  Value=0
  Constant{2..5,9} (5 alike) : Constant  Value=0  OutDataTypeStr=boolean
  Constant6 : Constant
  Constant7 : Constant  Value=0.001
  Constant8 : Constant
  Gain{,1..4} (5 alike) : Gain  Gain=1/3
  MATLAB Function : MATLAB Function  TreatAsAtomicUnit=on
  Product{1..41} (41 alike) : Product
  Programmable Pulse Generator : Subsystem
  S-R Flip-Flop{1..5} (5 alike) : simulink_extras/Flip Flops/S-R Flip-Flop  initial_condition=1
  Scope1 : Scope  NumInputPorts=5
  Step : Step  Time=0.5  SampleTime=0
  Subtract{1..20} (20 alike) : Sum  Inputs=+-
  Terminator{,1..4} (5 alike) : Terminator
  To File : ToFile  Filename=I_dc12  MatrixName=I_dc12
  To File1 : ToFile  Filename=I_dc21  MatrixName=I_dc21
  To File10 : ToFile  Filename=I_dc43  MatrixName=I_dc43
  To File2 : ToFile  Filename=I_dc23  MatrixName=I_dc23
  To File3 : ToFile  Filename=I_dc32  MatrixName=I_dc2
  To File5 : ToFile  Filename=I_dc14  MatrixName=I_dc14
  To File6 : ToFile  Filename=I_dc41  MatrixName=I_dc41
  To File7 : ToFile  Filename=I_dc24  MatrixName=I_dc24
  To File8 : ToFile  Filename=I_dc42  MatrixName=I_dc2
  To File9 : ToFile  Filename=I_dc34  MatrixName=I_dc34
  To Workspace : ToWorkspace  VariableName=I_dc12  SampleTime=-1
  To Workspace1 : ToWorkspace  VariableName=I_dc21  SampleTime=-1
  To Workspace10 : ToWorkspace  VariableName=I_dc43  SampleTime=-1
  To Workspace2 : ToWorkspace  VariableName=I_dc23  SampleTime=-1
  To Workspace3 : ToWorkspace  VariableName=I_dc32  SampleTime=-1
  To Workspace5 : ToWorkspace  VariableName=I_dc4  SampleTime=-1
  To Workspace6 : ToWorkspace  VariableName=I_dc41  SampleTime=-1
  To Workspace7 : ToWorkspace  VariableName=I_dc24  SampleTime=-1
  To Workspace8 : ToWorkspace  VariableName=I_dc42  SampleTime=-1
  To Workspace9 : ToWorkspace  VariableName=I_dc34  SampleTime=-1
  Transport Delay{1..20} (20 alike) : TransportDelay  DelayTime=0.001
  XOR{1..5} (5 alike) : Logic  Operator=NOT  Inputs=1  AllPortsSameDT=off  OutDataTypeStr=boolean
  di/dt OF DC CURRENT AT BUS {1..20} (20 alike) : Scope
  i012 1 : Scope
  i014 : Scope
  i021 2 : Scope
  i023 : Scope
  i024 : Scope
  i032 : Scope
  i034 : Scope
  i041 : Scope
  i042 : Scope
  i043 : Scope
  i{12,14,21,23..24,32,34,41..43} (10 alike) : Scope
  tag scope: tr12=global, tr14=global, tr23=global, tr24=global, tr34=global
  wires:
  [I0_dc34] -> i034/1
  [I_dc34] -> i34/1, To Workspace9/1, To File9/1
  [I_dc42] -> i42/1, To File8/1, To Workspace8/1
  [I_dc24] -> i24/1, To Workspace7/1, To File7/1
  [I0_dc24] -> i024/1
  [I0_dc32] -> i032/1
  [I0_dc42] -> i042/1
  [I0_dc14] -> i014/1
  [I_dc41] -> i41/1, To File6/1, To Workspace6/1
  [I0_dc23] -> i023/1
  [I_dc12] -> i12/1, To Workspace/1, To File/1
  [I_dc21] -> i21/1, To File1/1, To Workspace1/1
  [I0_dc43] -> i043/1
  MATLAB Function/4(tr23) -> XOR3/1
  S-R Flip-Flop4/1 -> Scope1/1, [tr12]  "tr12"
  [I_dc14] -> i14/1, To Workspace5/1, To File5/1
  MATLAB Function/3(tr24) -> XOR2/1
  [I0_dc21] -> i021 2/1
  S-R Flip-Flop1/2 -> Terminator1/1
  [I0_dc12] -> i012 1/1
  Constant8/1 -> Programmable Pulse Generator/3(PulseWidth)
  [I_dc43] -> i43/1, To File10/1, To Workspace10/1
  Constant4/1 -> S-R Flip-Flop3/1
  Programmable Pulse Generator/1(Pulse) -> Product9/1
  Constant9/1 -> S-R Flip-Flop5/1
  S-R Flip-Flop4/2 -> Terminator3/1
  MATLAB Function/1(tr12) -> XOR4/1
  [I_dc32] -> i32/1, To File3/1, To Workspace3/1
  XOR1/1 -> S-R Flip-Flop2/2
  [I_dc23] -> i23/1, To Workspace2/1, To File2/1
  XOR3/1 -> S-R Flip-Flop3/2
  Constant3/1 -> S-R Flip-Flop2/1
  XOR5/1 -> S-R Flip-Flop5/2
  Constant6/1 -> Programmable Pulse Generator/1(Amplitude)
  S-R Flip-Flop5/1 -> Scope1/5, [tr34]  "tr34"
  [I0_dc41] -> i041/1
  XOR4/1 -> S-R Flip-Flop4/2
  XOR2/1 -> S-R Flip-Flop1/2
  Constant2/1 -> S-R Flip-Flop1/1
  MATLAB Function/5(tr34) -> XOR5/1
  S-R Flip-Flop2/2 -> Terminator/1
  Constant5/1 -> S-R Flip-Flop4/1
  S-R Flip-Flop3/1 -> Scope1/4, [tr23]  "tr23"
  S-R Flip-Flop5/2 -> Terminator4/1
  S-R Flip-Flop2/1 -> Scope1/2, [tr14]  "tr14"
  S-R Flip-Flop1/1 -> [tr24], Scope1/3  "tr24"
  S-R Flip-Flop3/2 -> Terminator2/1
  Constant1/1 -> Programmable Pulse Generator/4(PhaseDelay)
  Product9/1 -> [trim]
  MATLAB Function/2(tr14) -> XOR1/1
  Step/1 -> Product9/2
  Constant7/1 -> Programmable Pulse Generator/2(Period)
  [I0_dc12] -> Product5/2, Transport Delay3/1
  Product5/1 -> Subtract3/1
  Subtract1/1 -> [dt12], di/dt OF DC CURRENT AT BUS 1/1  "signal 1"
  Transport Delay4/1 -> Product8/2
  Product3/1 -> Subtract1/2
  Product6/1 -> Subtract3/2
  Product4/1 -> Subtract2/2
  Product2/1 -> Subtract1/1
  Product1/1 -> Subtract2/1
  [trim] -> Product8/1, Product7/1
  Transport Delay2/1 -> Product4/2
  Transport Delay1/1 -> Product3/2
  [trim] -> Product4/1, Product1/1
  [I_dc21] -> Product1/2, Transport Delay2/1
  [trim] -> Product2/1, Product3/1
  [I0_dc21] -> Product7/2, Transport Delay4/1
  Product7/1 -> Subtract4/1
  [trim] -> Product6/1, Product5/1
  Subtract2/1 -> di/dt OF DC CURRENT AT BUS 2/1, [dt21]  "signal 2"
  [I_dc12] -> Product2/2, Transport Delay1/1
  Product8/1 -> Subtract4/2
  Gain/1 -> [dt021], di/dt OF DC CURRENT AT BUS 4/1
  Transport Delay3/1 -> Product6/2
  Subtract4/1 -> Gain/1  "signal 4"
  Subtract3/1 -> [dt012], di/dt OF DC CURRENT AT BUS 3/1  "signal 3"
  [dt12] -> MATLAB Function/1(dt12)
  [dt21] -> MATLAB Function/2(dt21)
  [dt012] -> MATLAB Function/3(dt012)
  [dt021] -> MATLAB Function/4(dt021)
  [I_dc32] -> Product10/2, Transport Delay6/1
  Transport Delay5/1 -> Product12/2
  Transport Delay6/1 -> Product13/2
  Product15/1 -> Subtract7/2
  Product10/1 -> Subtract6/1
  Product11/1 -> Subtract5/1
  [trim] -> Product17/1, Product16/1
  Transport Delay8/1 -> Product17/2
  [trim] -> Product13/1, Product10/1
  Product12/1 -> Subtract5/2
  Subtract8/1 -> Gain1/1  "signal 4"
  [I0_dc23] -> Product14/2, Transport Delay7/1
  Transport Delay7/1 -> Product15/2
  Product17/1 -> Subtract8/2
  Subtract7/1 -> [dt023], di/dt OF DC CURRENT AT BUS 7/1  "signal 3"
  Product13/1 -> Subtract6/2
  [I_dc23] -> Product11/2, Transport Delay5/1
  Subtract6/1 -> di/dt OF DC CURRENT AT BUS 6/1, [dt32]  "signal 2"
  Gain1/1 -> [dt032], di/dt OF DC CURRENT AT BUS 8/1
  Product16/1 -> Subtract8/1
  Subtract5/1 -> [dt23], di/dt OF DC CURRENT AT BUS 5/1  "signal 1"
  [I0_dc32] -> Product16/2, Transport Delay8/1
  Product14/1 -> Subtract7/1
  [trim] -> Product11/1, Product12/1
  [trim] -> Product15/1, Product14/1
  [I_dc41] -> Product18/2, Transport Delay10/1
  Transport Delay9/1 -> Product20/2
  Transport Delay10/1 -> Product21/2
  Product23/1 -> Subtract11/2
  Product18/1 -> Subtract10/1
  Product19/1 -> Subtract9/1
  [trim] -> Product25/1, Product24/1
  Transport Delay12/1 -> Product25/2
  [trim] -> Product21/1, Product18/1
  Product20/1 -> Subtract9/2
  Subtract12/1 -> Gain2/1  "signal 4"
  [I0_dc14] -> Product22/2, Transport Delay11/1
  Transport Delay11/1 -> Product23/2
  Product25/1 -> Subtract12/2
  Subtract11/1 -> [dt014], di/dt OF DC CURRENT AT BUS 11/1  "signal 3"
  Product21/1 -> Subtract10/2
  [I_dc14] -> Product19/2, Transport Delay9/1
  Subtract10/1 -> di/dt OF DC CURRENT AT BUS 10/1, [dt41]  "signal 2"
  Gain2/1 -> [dt041], di/dt OF DC CURRENT AT BUS 12/1
  Product24/1 -> Subtract12/1
  Subtract9/1 -> [dt14], di/dt OF DC CURRENT AT BUS 9/1  "signal 1"
  [I0_dc41] -> Product24/2, Transport Delay12/1
  Product22/1 -> Subtract11/1
  [trim] -> Product19/1, Product20/1
  [trim] -> Product23/1, Product22/1
  [I_dc42] -> Product26/2, Transport Delay14/1
  Transport Delay13/1 -> Product28/2
  Transport Delay14/1 -> Product29/2
  Product31/1 -> Subtract15/2
  Product26/1 -> Subtract14/1
  Product27/1 -> Subtract13/1
  [trim] -> Product33/1, Product32/1
  Transport Delay16/1 -> Product33/2
  [trim] -> Product29/1, Product26/1
  Product28/1 -> Subtract13/2
  Subtract16/1 -> Gain3/1  "signal 4"
  [I0_dc24] -> Product30/2, Transport Delay15/1
  Transport Delay15/1 -> Product31/2
  Product33/1 -> Subtract16/2
  Subtract15/1 -> [dt024], di/dt OF DC CURRENT AT BUS 15/1  "signal 3"
  Product29/1 -> Subtract14/2
  [I_dc24] -> Product27/2, Transport Delay13/1
  Subtract14/1 -> di/dt OF DC CURRENT AT BUS 14/1, [dt42]  "signal 2"
  Gain3/1 -> [dt042], di/dt OF DC CURRENT AT BUS 16/1
  Product32/1 -> Subtract16/1
  Subtract13/1 -> [dt24], di/dt OF DC CURRENT AT BUS 13/1  "signal 1"
  [I0_dc42] -> Product32/2, Transport Delay16/1
  Product30/1 -> Subtract15/1
  [trim] -> Product27/1, Product28/1
  [trim] -> Product31/1, Product30/1
  [I_dc43] -> Product34/2, Transport Delay18/1
  Transport Delay17/1 -> Product36/2
  Transport Delay18/1 -> Product37/2
  Product39/1 -> Subtract19/2
  Product34/1 -> Subtract18/1
  Product35/1 -> Subtract17/1
  [trim] -> Product41/1, Product40/1
  Transport Delay20/1 -> Product41/2
  [trim] -> Product37/1, Product34/1
  Product36/1 -> Subtract17/2
  Subtract20/1 -> Gain4/1  "signal 4"
  [I0_dc34] -> Product38/2, Transport Delay19/1
  Transport Delay19/1 -> Product39/2
  Product41/1 -> Subtract20/2
  Subtract19/1 -> [dt034], di/dt OF DC CURRENT AT BUS 19/1  "signal 3"
  Product37/1 -> Subtract18/2
  [I_dc34] -> Product35/2, Transport Delay17/1
  Subtract18/1 -> di/dt OF DC CURRENT AT BUS 18/1, [dt43]  "signal 2"
  Gain4/1 -> [dt043], di/dt OF DC CURRENT AT BUS 20/1
  Product40/1 -> Subtract20/1
  Subtract17/1 -> [dt34], di/dt OF DC CURRENT AT BUS 17/1  "signal 1"
  [I0_dc43] -> Product40/2, Transport Delay20/1
  Product38/1 -> Subtract19/1
  [trim] -> Product35/1, Product36/1
  [trim] -> Product39/1, Product38/1
  [dt043] -> MATLAB Function/20(dt043)
  [dt23] -> MATLAB Function/5(dt23)
  [dt32] -> MATLAB Function/6(dt32)
  [dt023] -> MATLAB Function/7(dt023)
  [dt032] -> MATLAB Function/8(dt032)
  [dt14] -> MATLAB Function/9(dt14)
  [dt41] -> MATLAB Function/10(dt41)
  [dt014] -> MATLAB Function/11(dt014)
  [dt041] -> MATLAB Function/12(dt041)
  [dt24] -> MATLAB Function/13(dt24)
  [dt42] -> MATLAB Function/14(dt42)
  [dt024] -> MATLAB Function/15(dt024)
  [dt042] -> MATLAB Function/16(dt042)
  [dt34] -> MATLAB Function/17(dt34)
  [dt43] -> MATLAB Function/18(dt43)
  [dt034] -> MATLAB Function/19(dt034)

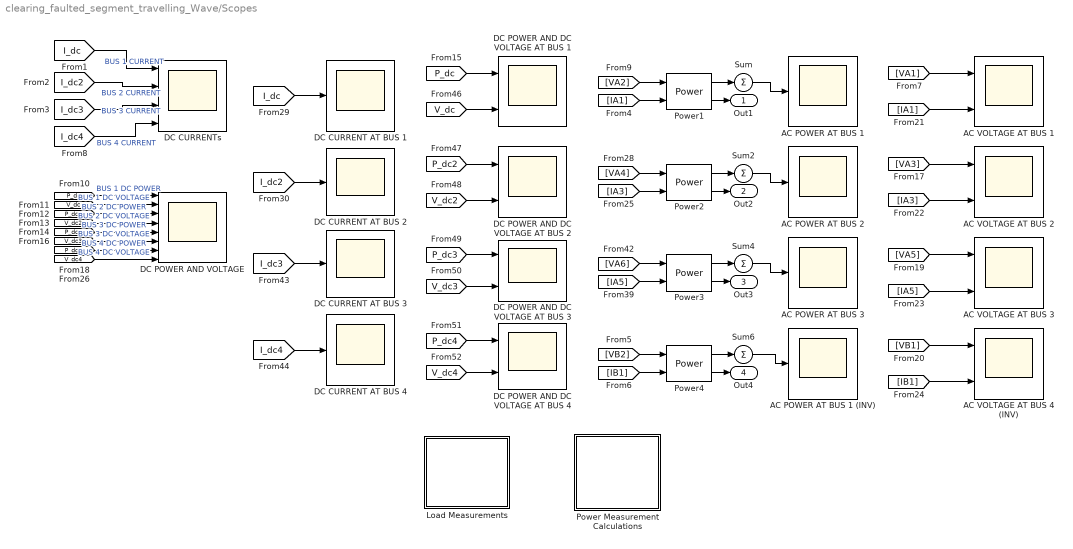
== system clearing_faulted_segment_travelling_Wave/Scopes  ==
  AC POWER AT BUS 1 : Scope
  AC POWER AT BUS 1 (INV) : Scope
  AC POWER AT BUS 2 : Scope
  AC POWER AT BUS 3 : Scope
  AC VOLTAGE AT BUS 1 : Scope  NumInputPorts=2
  AC VOLTAGE AT BUS 2 : Scope  NumInputPorts=2
  AC VOLTAGE AT BUS 3 : Scope  NumInputPorts=2
  AC VOLTAGE AT BUS 4 (INV) : Scope  NumInputPorts=2
  DC CURRENT AT BUS {1..4} (4 alike) : Scope
  DC CURRENTs : Scope  NumInputPorts=4
  DC POWER AND DC VOLTAGE AT BUS {1..4} (4 alike) : Scope  NumInputPorts=2
  DC POWER AND VOLTAGE : Scope  NumInputPorts=8
  "Load Measurements " : Subsystem
  Power Measurement Calculations : Subsystem
  Power{1..4} (4 alike) : powerlib_meascontrol/Measurements/Power  Freq=f  Vinit=[1, 0]  Iinit=[1, 0]  Ts=0
      settings: SourceProductName=Simscape Electrical
  Sum{,2,4,6} (4 alike) : Sum  Inputs=1
  Out1 : Outport
  Out2 : Outport  Port=2
  Out3 : Outport  Port=3
  Out4 : Outport  Port=4
  wires:
  Sum6/1 -> AC POWER AT BUS 1 (INV)/1
  [I_dc] -> DC CURRENT AT BUS 1/1
  Power2/2 -> Out2/1
  [IA1] -> Power1/2
  [IA3] -> AC VOLTAGE AT BUS 2/2
  [IB1] -> Power4/2
  Sum/1 -> AC POWER AT BUS 1/1
  [IB1] -> AC VOLTAGE AT BUS 4 (INV)/2
  [VA4] -> Power2/1
  [I_dc4] -> DC CURRENT AT BUS 4/1
  [V_dc2] -> DC POWER AND DC VOLTAGE AT BUS 2/2
  Power1/1 -> Sum/1
  [VA6] -> Power3/1
  Power1/2 -> Out1/1
  Power4/1 -> Sum6/1
  [IA5] -> AC VOLTAGE AT BUS 3/2
  [I_dc2] -> DC CURRENT AT BUS 2/1
  [I_dc3] -> DC CURRENT AT BUS 3/1
  [VA1] -> AC VOLTAGE AT BUS 1/1
  [IA1] -> AC VOLTAGE AT BUS 1/2
  [VA2] -> Power1/1
  Power3/1 -> Sum4/1
  [VB2] -> Power4/1
  [IA3] -> Power2/2
  [IA5] -> Power3/2
  [V_dc] -> DC POWER AND DC VOLTAGE AT BUS 1/2
  [P_dc4] -> DC POWER AND DC VOLTAGE AT BUS 4/1
  [V_dc3] -> DC POWER AND DC VOLTAGE AT BUS 3/2
  [P_dc2] -> DC POWER AND DC VOLTAGE AT BUS 2/1
  [V_dc4] -> DC POWER AND DC VOLTAGE AT BUS 4/2
  Power4/2 -> Out4/1
  Power2/1 -> Sum2/1
  [P_dc3] -> DC POWER AND DC VOLTAGE AT BUS 3/1
  [P_dc] -> DC POWER AND DC VOLTAGE AT BUS 1/1
  Sum4/1 -> AC POWER AT BUS 3/1
  [VA3] -> AC VOLTAGE AT BUS 2/1
  [VB1] -> AC VOLTAGE AT BUS 4 (INV)/1
  [VA5] -> AC VOLTAGE AT BUS 3/1
  Sum2/1 -> AC POWER AT BUS 2/1
  Power3/2 -> Out3/1
  [I_dc] -> DC CURRENTs/1  "BUS 1 CURRENT"
  [I_dc2] -> DC CURRENTs/2  "BUS 2 CURRENT"
  [I_dc3] -> DC CURRENTs/3  "BUS 3 CURRENT"
  [I_dc4] -> DC CURRENTs/4  "BUS 4 CURRENT"
  [P_dc] -> DC POWER AND VOLTAGE/1  "BUS 1 DC POWER"
  [V_dc] -> DC POWER AND VOLTAGE/2  "BUS 1 DC VOLTAGE"
  [P_dc2] -> DC POWER AND VOLTAGE/3  "BUS 2 DC POWER"
  [V_dc2] -> DC POWER AND VOLTAGE/4  "BUS 2 DC VOLTAGE"
  [P_dc3] -> DC POWER AND VOLTAGE/5  "BUS 3 DC POWER"
  [V_dc3] -> DC POWER AND VOLTAGE/6  "BUS 3 DC VOLTAGE"
  [P_dc4] -> DC POWER AND VOLTAGE/7  "BUS 4 DC POWER"
  [V_dc4] -> DC POWER AND VOLTAGE/8  "BUS 4 DC VOLTAGE"
